simulink model "DCMotorModel"  (R2024b)
settings: Solver=FixedStepAuto  StartTime=0.0  StopTime=10  FixedStep=0.1  RelTol=1e-3
values from neighbouring files (symbols this model uses):
  B = 6.09e-5    (= 6.09e-05)    [dc_motor_simulink_setup.m]
  J = 5.7e-7    (= 5.7e-07)    [dc_motor_simulink_setup.m]
  Ke = 0.00109    [dc_motor_simulink_setup.m]
  Kt = 0.0104    [dc_motor_simulink_setup.m]
  La = 1.19e-4    (= 0.000119)    [dc_motor_simulink_setup.m]
  Ra = 1.6    [dc_motor_simulink_setup.m]
libraries: simulink x1
settings Model: Creator=nps22  LastModifiedBy=nps22

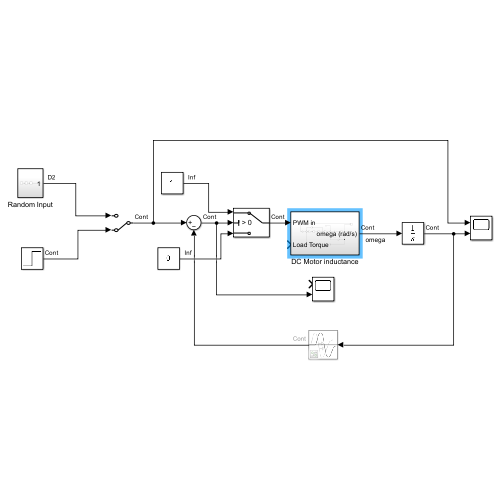
[thumbnail: Simulink's stored preview of the top-level diagram]
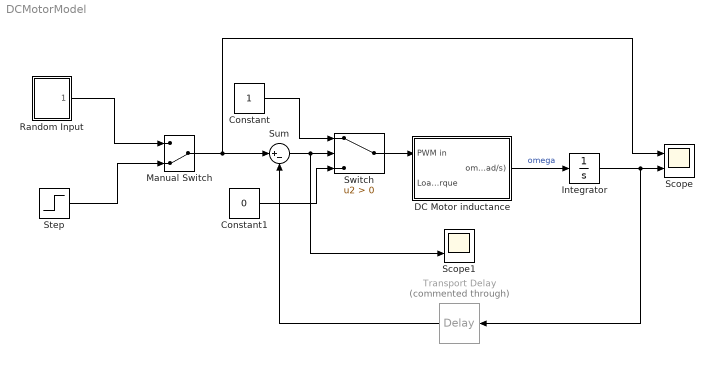
== system DCMotorModel ==
  Constant : Constant
  Constant1 : Constant  Value=0
  DC Motor inductance : Subsystem
  Integrator : Integrator
  Manual Switch : ManualSwitch  CurrentSetting=0
  Random Input : Subsystem
  Scope : Scope  NumInputPorts=2
  Scope1 : Scope  NumInputPorts=2
  Step : Step  After=1000  SampleTime=0
  Sum : Sum  Inputs=|+-
  Switch : Switch  Criteria=u2 > Threshold  SaturateOnIntegerOverflow=off  InputSameDT=off
  Transport Delay : TransportDelay  Commented=through  DelayTime=0.01
  wires:
  DC Motor inductance/1(omega (rad/s)) -> Integrator/1  "omega"
  Sum/1 -> Switch/2, Scope1/2
  Manual Switch/1 -> Scope/1, Sum/1
  Random Input/1(Out1) -> Manual Switch/1
  Step/1 -> Manual Switch/2
  Transport Delay/1 -> Sum/2
  Integrator/1 -> Transport Delay/1, Scope/2
  Switch/1 -> DC Motor inductance/1(PWM in)
  Constant/1 -> Switch/1
  Constant1/1 -> Switch/3

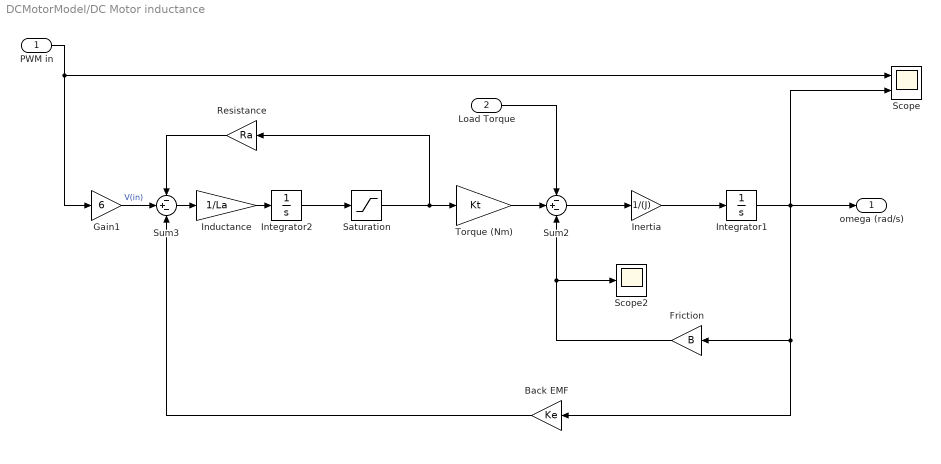
== system DCMotorModel/DC Motor inductance ==
  PWM in : Inport
  Load Torque : Inport  Port=2
  Back EMF : Gain  Gain=Ke
  Friction : Gain  Gain=B
  Gain1 : Gain  Gain=6
  Inductance : Gain  Gain=1/La
  Inertia : Gain  Gain=1/(J)
  Integrator1 : Integrator
  Integrator2 : Integrator
  Resistance : Gain  Gain=Ra
  Saturation : Saturate  UpperLimit=1  LowerLimit=-1
  Scope : Scope  NumInputPorts=2
  Scope2 : Scope
  Sum2 : Sum  Inputs=-+-
  Sum3 : Sum  Inputs=-+-
  Torque (Nm) : Gain  Gain=Kt
  omega (rad/s) : Outport
  wires:
  Back EMF/1 -> Sum3/3
  Resistance/1 -> Sum3/1
  Inertia/1 -> Integrator1/1
  Integrator2/1 -> Saturation/1
  Sum3/1 -> Inductance/1
  Friction/1 -> Sum2/3, Scope2/1
  Sum2/1 -> Inertia/1
  Integrator1/1 -> Scope/2, omega (rad/s)/1, Friction/1, Back EMF/1
  Inductance/1 -> Integrator2/1
  Torque (Nm)/1 -> Sum2/2
  Load Torque/1 -> Sum2/1
  Gain1/1 -> Sum3/2  "V(in)"
  PWM in/1 -> Gain1/1, Scope/1
  Saturation/1 -> Resistance/1, Torque (Nm)/1

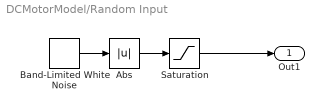
== system DCMotorModel/Random Input ==
  Abs : Abs  SaturateOnIntegerOverflow=off
  Band-Limited White Noise : simulink/Sources/Band-Limited White Noise  Cov=[3e4]  Ts=1  seed=[23341]
  Saturation : Saturate  UpperLimit=350  LowerLimit=0
  Out1 : Outport
  wires:
  Abs/1 -> Saturation/1
  Band-Limited White Noise/1 -> Abs/1
  Saturation/1 -> Out1/1
